simulink library "tqd"  (R2021b)
settings: Solver=VariableStepAuto  StartTime=0.0  StopTime=10.0  RelTol=1e-3
undefined symbols (not defined in the file or in its folder): ATQD_APSDecReq_X_kph, ATQD_APSDecReq_Y_mps2, ATQD_APSDecReqCMD_X_kph, ATQD_APSDecReqTs_X_pct, ATQD_APSDecTimeGain_X_Deg, ATQD_APSDecTimeGain_Y_s, ATQD_APSReqLowSpd_X_Deg, ATQD_AutoHoldReleaseBPS_X_Deg, ATQD_AWDLoadTrqnsGain_X_kg, ATQD_AWDLoadTrqnsGain_Y_pct, ATQD_BOSEnBPSPosn_X_kph, ATQD_BOSMap_X_rpm, ATQD_BOSMap_Y_pct, ATQD_CreepBaseTqD_X_kph, ATQD_CreepBaseTqD_Y_Deg, ATQD_CreepBaseTqR_X_kph, ATQD_CreepBaseTqR_Y_Deg, ATQD_CreepBPSDisPosn_X_Deg, ATQD_CreepBPSDisPosnR_X_Deg, ATQD_CreepBPSEnPosn_X_Deg, ATQD_CreepBPSEnPosnR_X_Deg, ATQD_CreepDeltaTq_X_kph, ATQD_CreepIterm_X_kph, ATQD_CreepIterm_Y_kph, ATQD_CreepItermMaxLimit_X_pct, ATQD_CreepPreloadTime_X_kph, ATQD_CreepPreloadTq_X_kph, ATQD_CreepPreloadTq_Y_s, ATQD_CreepProtTq_X_Deg, ATQD_CreepPterm_X_kph, ATQD_ECOTqMapD_X_rpm, ATQD_ECOTqMapD_Y_pct, ATQD_EOPDTqMapDCon_X_rpm, ATQD_EOPDTqMapDCon_Y_Deg, ATQD_EstInitVehWeight_X_c, ATQD_LHMRollGenMapD_X_rpm, ATQD_LHMRollGenMapD_Y_rpm, ATQD_LHMTqMapD_X_rpm, ATQD_LHMTqMapD_Y_pct, ATQD_NL1TqMapD_X_rpm, ATQD_NL1TqMapD_Y_pct, ATQD_NOPDTqMapDCon_X_rpm, ATQD_NOPDTqMapDCon_Y_Deg, ATQD_NRMRrEDUSpRat_X_rpm, ATQD_NRMRrEDUSpRat_Y_Nm, ATQD_OPDHoldDownRelDelay_X_Deg, ATQD_OPDHoldEnSpd_X_Deg, ATQD_OPDHoldRelDetTime_X_Deg, ATQD_OPDHoldReleaseTq_X_Deg, ATQD_OrigPedTqLowLim_X_Deg, ATQD_OrigPedTqLowLim_Y_pct, ATQD_PedalMapClimbUpLim_X_rpm, ATQD_PedalMapClimbUpLim_Y_Deg, ATQD_PreLoadTq_X_s, ATQD_RollGenMapEL1_X_rpm, ATQD_RollGenMapEL1_Y_rpm, ATQD_SL1TqMapD_X_rpm, ATQD_SL1TqMapD_Y_pct, ATQD_SlideRegenTqGain_X_Gps, ATQD_SlideRegenTqGain_Y_pct ... (+378)
libraries: hcu_lib x59, simulink x49
(part 8 of 12)

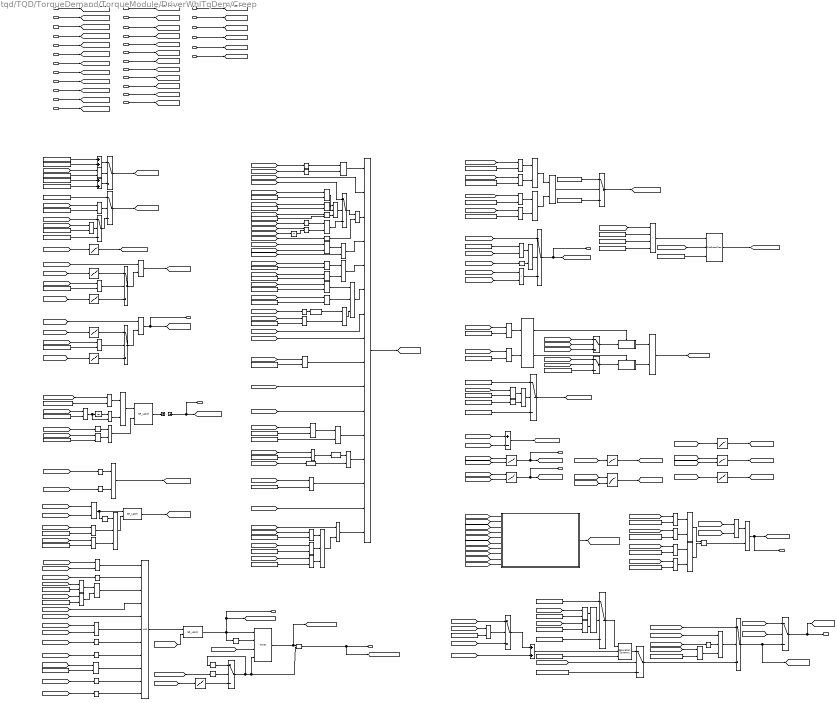
== system tqd/TQD/TorqueDemand/TorqueModule/DriverWhlTqDem/Creep ==
  note: Creep Wheel Torque Demand Calculation
  note: Vehicle Actual Speed Calculation
  note: Creep Enable Judgement
  VTQD_CreepON_flg : Inport
  VTQD_GearActualPosn_enum : Inport  Port=2
  VTQD_LowIdleAccPedal_flg : Inport  Port=3
  VINP_VehSpeed_kph : Inport  Port=4
  VTQD_TMRotateDirction_enum : Inport  Port=5
  VTQD_RegenMode_enum : Inport  Port=6
  VTQD_ActBPSPosn_pct : Inport  Port=7
  VTQD_PedalMapWhlTq_Nm : Inport  Port=8
  VINP_RrRBCActive_flg : Inport  Port=9
  VINP_FrRBCActive_flg : Inport  Port=10
  VVMC_ADASActive_flg : Inport  Port=11
  task_time_s : Inport  Port=12
  VTQD_LoSpdBrkCtrl_flg : Inport  Port=13
  VINP_AVHActive_flg : Inport  Port=14
  VTQD_APSReq_enum : Inport  Port=15
  VVMC_APSSpeedCMD_kph : Inport  Port=16
  VVMC_APSActive_flg : Inport  Port=17
  VTQD_RDCActive_enum : Inport  Port=18
  VVMC_APSReq_enum : Inport  Port=19
  " VINP_FrEDURealTMTq_Nm" : Inport  Port=20
  VINP_RrEDURealTMTq_Nm : Inport  Port=21
  VTQD_PreLoadPreEn_flg : Inport  Port=22
  VVMC_EstSlope_Deg : Inport  Port=23
  VPMM_PwrSta_enum : Inport  Port=24
  VTQD_TqTargetShaftSpd_rpm : Inport  Port=25
  VTQD_APSReqTimer_s : Inport  Port=26
  VINP_EPBSta_enum : Inport  Port=27
  VTQD_OPDHoldEnRel_flg : Inport  Port=28
  VTQD_ActAPSPosn_pct : Inport  Port=29
  VVMC_CAASActive_flg : Inport  Port=30
  AND{,1..2,4..7,9,11..13,15} (12 alike) : Logic  AllPortsSameDT=off  OutDataTypeStr=boolean
  AND10 : Logic  Operator=OR  AllPortsSameDT=off  OutDataTypeStr=boolean
  AND14 : Logic  Inputs=3  AllPortsSameDT=off  OutDataTypeStr=boolean
  AND3 : Logic  Inputs=3  AllPortsSameDT=off  OutDataTypeStr=boolean
  AND8 : Logic  Inputs=3  AllPortsSameDT=off  OutDataTypeStr=boolean
  Add : Sum  Inputs=+-
  Add1 : Sum
  Add2 : Sum
  Add4 : Sum
  Constant1 : Constant  Value=KTQD_APSCMDEnCreepSpd_kph
  Constant10 : Constant  Value=KTQD_CreepTargetSpdR_kph
  Constant{3,11..12,21,25,58,62} (7 alike) : Constant  Value=ENUM_GEARACTUALPOSN_D
  Constant13 : Constant  Value=KTQD_CreepEnableSpd_kph
  Constant14 : Constant  Value=RPM2RADPS
  Constant15 : Constant  Value=ZERO_FLOAT
  Constant16 : Constant  Value=KTQD_TireRadius_m
  Constant17 : Constant  Value=ENUM_RDCACTSTA_NOREQUEST
  Constant18 : Constant  Value=ENUM_APSREQ_DECELCTRL  OutDataTypeStr=uint8
  Constant19 : Constant  Value=MPS2KPH
  Constant{2,9,20,31,35..36,38,42..44} (10 alike) : Constant  Value=ENUM_GEARACTUALPOSN_R
  Constant22 : Constant  Value=KTQD_CreepLowLimitTq_Nm
  Constant23 : Constant  Value=KTQD_CreepPrLoadEnSpd_kph
  Constant24 : Constant  Value=ENUM_RDCACTSTA_NOREQUEST
  Constant26 : Constant  Value=KTQD_CreepDisableSpdofst_kph
  Constant27 : Constant  Value=KTQD_CreepEnableSpdR_kph
  Constant28 : Constant  Value=KTQD_CreepDisableSpdofstR_kph
  Constant29 : Constant  Value=KTQD_CreepEnableSpdR_kph
  Constant30 : Constant  Value=ENUM_TMROTATEDIRECTACT_REVERSE  OutDataTypeStr=Inherit: Inherit via back propagation
  Constant32 : Constant  Value=ENUM_TMROTATEDIRECTACT_FORWARD  OutDataTypeStr=Inherit: Inherit via back propagation
  Constant33 : Constant  Value=KTQD_VehActSpdNegGain_gain
  Constant34 : Constant  Value=KTQD_VehActSpdPosGain_gain
  Constant37 : Constant  Value=ENUM_TMROTATEDIRECTACT_REVERSE  OutDataTypeStr=Inherit: Inherit via back propagation
  Constant39 : Constant  Value=ENUM_TMROTATEDIRECTACT_FORWARD  OutDataTypeStr=Inherit: Inherit via back propagation
  Constant{4,8,52,54,59,64} (6 alike) : Constant  Value=ENUM_REGENLEVEL_OPD
  Constant40 : Constant  Value=KTQD_RBCCreepRecTq_Nm
  Constant41 : Constant  Value=KTQD_RBCCreepRecTq_Nm
  Constant45 : Constant  Value=ENUM_POWERSTA_READY
  Constant46 : Constant  Value=KTQD_CreepEnableSpd_kph
  Constant47 : Constant  Value=KTQD_RPM2VehSpdTs_c
  Constant48 : Constant  Value=KTQD_CreepVehSpdSW_flg
  Constant49 : Constant  Value=KTQD_CreepTargetSpdD_kph
  Constant5 : Constant  Value=ENUM_APSREQ_BRKHOLD  OutDataTypeStr=uint8
  Constant50 : Constant  Value=KTQD_OPDCreepTargetSpdD_kph
  Constant51 : Constant  Value=KTQD_APSReqDisCreep_flg  OutDataTypeStr=uint8
  Constant53 : Constant  Value=KTQD_APSReqDelayTime_s
  Constant55 : Constant  Value=ENUM_EPBSTA_APPLIED  OutDataTypeStr=uint8
  Constant56 : Constant  Value=KTQD_APSReqDisCreep_flg
  Constant57 : Constant  Value=KTQD_CreepUpLimitTq_Nm
  Constant6 : Constant  Value=ENUM_GEARACTUALPOSN_P
  Constant60 : Constant  Value=KTQD_OPDCreepDUpLimitTq_Nm
  Constant61 : Constant  Value=KTQD_CreepDisPedTqSpd_kph
  Constant63 : Constant  Value=KTQD_CreepAPSPosn2Launch_pct
  Constant65 : Constant  Value=ENUM_APSREQ_DECELCTRL  OutDataTypeStr=uint8
  Constant7 : Constant  Value=ENUM_GEARACTUALPOSN_N
  Data Type Conversion : DataTypeConversion
  Delay : Delay  DelayLength=1
  Delay1 : Delay  DelayLength=1
  Detect Change : simulink/Logic and Bit Operations/Detect Change  vinit=0  OutDataTypeStr=boolean
  Detect Increase : simulink/Logic and Bit Operations/Detect Increase  vinit=0.0  OutDataTypeStr=boolean
  Equal{,1..4,6..8,10..16,19..31,33..39} (35 alike) : RelationalOperator  Operator===  OutDataTypeStr=boolean  RndMeth=Simplest
  Equal17 : RelationalOperator  Operator=<=  OutDataTypeStr=boolean  RndMeth=Simplest
  Equal18 : RelationalOperator  Operator=~=  OutDataTypeStr=boolean  RndMeth=Simplest
  Equal32 : RelationalOperator  OutDataTypeStr=boolean  RndMeth=Simplest
  Equal5 : RelationalOperator  Operator=<=  OutDataTypeStr=boolean  RndMeth=Simplest
  Equal9 : RelationalOperator  Operator=<=  OutDataTypeStr=boolean  RndMeth=Simplest
  FirstOrderFilter : hcu_lib/Basic_Blocks/FirstOrderFilter
  GreaterThan : RelationalOperator  Operator=>  OutDataTypeStr=boolean  RndMeth=Simplest
  GreaterThan1 : RelationalOperator  Operator=>  OutDataTypeStr=boolean  RndMeth=Simplest
  GreaterThan2 : RelationalOperator  OutDataTypeStr=boolean  RndMeth=Simplest
  GreaterThan3 : RelationalOperator  Operator=>  OutDataTypeStr=boolean  RndMeth=Simplest
  GreaterThan4 : RelationalOperator  Operator=<=  OutDataTypeStr=boolean  RndMeth=Simplest
  Ground2 : Ground
  If : If  NumInputs=2  IfExpression=u1 ~= 0  ElseIfExpressions=u2 ~= 0  ShowElse=off
  If Action Subsystem : Subsystem  TreatAsAtomicUnit=on
  If Action Subsystem1 : Subsystem  TreatAsAtomicUnit=on
  LiuzgSwitch1 : Switch  Criteria=u2 ~= 0
      settings: AttributesFormatString=<%<Criteria>>
  Logical Operator{,2,4,6} (4 alike) : Logic  AllPortsSameDT=off  OutDataTypeStr=boolean
  Logical Operator1 : Logic  Operator=OR  AllPortsSameDT=off  OutDataTypeStr=boolean
  Logical Operator3 : Logic  Inputs=11  AllPortsSameDT=off  OutDataTypeStr=boolean
  Logical Operator5 : Logic  Operator=OR  AllPortsSameDT=off  OutDataTypeStr=boolean
  MTQD_CreepBPSDisPosnR_Y_pct : Lookup_n-D  NumberOfTableDimensions=1  BreakpointsForDimension1=ATQD_CreepBPSDisPosnR_X_Deg  Table=MTQD_CreepBPSDisPosnR_Y_pct  ExtrapMethod=Clip  InternalRulePriority=Speed  RndMeth=Simplest  InputSameDT=on
  MTQD_CreepBPSDisPosn_Y_pct : Lookup_n-D  NumberOfTableDimensions=1  BreakpointsForDimension1=ATQD_CreepBPSDisPosn_X_Deg  Table=MTQD_CreepBPSDisPosn_Y_pct  ExtrapMethod=Clip  InternalRulePriority=Speed  RndMeth=Simplest  InputSameDT=on
  MTQD_CreepBPSEnPosnR_Y_pct : Lookup_n-D  NumberOfTableDimensions=1  BreakpointsForDimension1=ATQD_CreepBPSEnPosnR_X_Deg  Table=MTQD_CreepBPSEnPosnR_Y_pct  ExtrapMethod=Clip  InternalRulePriority=Speed  RndMeth=Simplest  InputSameDT=on
  MTQD_CreepBPSEnPosn_Y_pct : Lookup_n-D  NumberOfTableDimensions=1  BreakpointsForDimension1=ATQD_CreepBPSEnPosn_X_Deg  Table=MTQD_CreepBPSEnPosn_Y_pct  ExtrapMethod=Clip  InternalRulePriority=Speed  RndMeth=Simplest  InputSameDT=on
  MTQD_CreepBaseTqD_Z_Nm : Lookup_n-D  BreakpointsForDimension1=ATQD_CreepBaseTqD_Y_Deg  BreakpointsForDimension2=ATQD_CreepBaseTqD_X_kph  Table=MTQD_CreepBaseTqD_Z_Nm  ExtrapMethod=Clip  InternalRulePriority=Speed  RndMeth=Simplest  InputSameDT=on
      settings: InputPortMap=u0,u1
  MTQD_CreepBaseTqR_Z_Nm : Lookup_n-D  BreakpointsForDimension1=ATQD_CreepBaseTqR_Y_Deg  BreakpointsForDimension2=ATQD_CreepBaseTqR_X_kph  Table=MTQD_CreepBaseTqR_Z_Nm  ExtrapMethod=Clip  InternalRulePriority=Speed  RndMeth=Simplest  InputSameDT=on
      settings: InputPortMap=u0,u1
  MTQD_CreepDeltaTq_Y_Nm : Lookup_n-D  NumberOfTableDimensions=1  BreakpointsForDimension1=ATQD_CreepDeltaTq_X_kph  Table=MTQD_CreepDeltaTq_Y_Nm  ExtrapMethod=Clip  InternalRulePriority=Speed  RndMeth=Simplest  InputSameDT=on
  MTQD_CreepIterm_Z_Nm : Lookup_n-D  BreakpointsForDimension1=ATQD_CreepIterm_Y_kph  BreakpointsForDimension2=ATQD_CreepIterm_X_kph  Table=MTQD_CreepIterm_Z_Nm  ExtrapMethod=Clip  InternalRulePriority=Speed  RndMeth=Simplest  InputSameDT=on
      settings: InputPortMap=u0,u1
  MTQD_CreepPrelaodTq_Z_Nm : Lookup_n-D  BreakpointsForDimension1=ATQD_CreepPreloadTq_Y_s  BreakpointsForDimension2=ATQD_CreepPreloadTq_X_kph  Table=MTQD_CreepPreloadTq_Z_Nm  ExtrapMethod=Clip  InternalRulePriority=Speed  RndMeth=Simplest  InputSameDT=on
      settings: InputPortMap=u0,u1
  MTQD_CreepPreloadTime_Y_s : Lookup_n-D  NumberOfTableDimensions=1  BreakpointsForDimension1=ATQD_CreepPreloadTime_X_kph  Table=MTQD_CreepPreloadTime_Y_s  ExtrapMethod=Clip  InternalRulePriority=Speed  RndMeth=Simplest  InputSameDT=on
  MTQD_CreepProtTq_Y_Nm : Lookup_n-D  NumberOfTableDimensions=1  BreakpointsForDimension1=ATQD_CreepProtTq_X_Deg  Table=MTQD_CreepProtTq_Y_Nm  ExtrapMethod=Clip  InternalRulePriority=Speed  RndMeth=Simplest  InputSameDT=on
  MTQD_CreepPterm_Y_c : Lookup_n-D  NumberOfTableDimensions=1  BreakpointsForDimension1=ATQD_CreepPterm_X_kph  Table=MTQD_CreepPterm_Y_Nm  ExtrapMethod=Clip  InternalRulePriority=Speed  RndMeth=Simplest  InputSameDT=on
  MTQD_OPDHoldEnSpd_Y_kph : Lookup_n-D  NumberOfTableDimensions=1  BreakpointsForDimension1=ATQD_OPDHoldEnSpd_X_Deg  Table=MTQD_OPDHoldEnSpd_Y_kph  ExtrapMethod=Clip  InternalRulePriority=Speed  RndMeth=Simplest  InputSameDT=on
  Merge : Merge
  NOT{,1..15} (16 alike) : Logic  Operator=NOT  AllPortsSameDT=off  OutDataTypeStr=boolean
  OR{,2..3,6..9} (7 alike) : Logic  Operator=OR  AllPortsSameDT=off  OutDataTypeStr=boolean
  OR1 : Logic  Operator=OR  Inputs=16  AllPortsSameDT=off  OutDataTypeStr=boolean
  OR4 : Logic  Inputs=3  AllPortsSameDT=off  OutDataTypeStr=boolean
  OR5 : Logic  Operator=OR  Inputs=3  AllPortsSameDT=off  OutDataTypeStr=boolean
  Product : Product
  Product1 : Product  Inputs=4
  Relational Operator : RelationalOperator  OutDataTypeStr=boolean  RndMeth=Simplest
  Relational Operator1 : RelationalOperator  Operator=<  OutDataTypeStr=boolean  RndMeth=Simplest
  Relational Operator2 : RelationalOperator  Operator=>  OutDataTypeStr=boolean  RndMeth=Simplest
  Relational Operator3 : RelationalOperator  Operator=>  OutDataTypeStr=boolean  RndMeth=Simplest
  Relational Operator4 : RelationalOperator  Operator=>  OutDataTypeStr=boolean  RndMeth=Simplest
  Relational Operator5 : RelationalOperator  Operator=<=  OutDataTypeStr=boolean  RndMeth=Simplest
  Relay : Relay  OnSwitchValue=KTQD_OPDCreepEnGrade_Deg  OffSwitchValue=KTQD_OPDCreepDisGrade_Deg  OnOutputValue=0  OffOutputValue=1
  Relay1 : Relay  OnSwitchValue=KTQD_CreepDisVehSpd_kph  OffSwitchValue=KTQD_CreepEnVehSpd_kph  OnOutputValue=0  OffOutputValue=1  OutDataTypeStr=boolean
  SR_Latch : hcu_lib/Basic_Blocks/SR_Latch
  SR_Latch1 : hcu_lib/Basic_Blocks/SR_Latch
  SR_Latch3 : hcu_lib/Basic_Blocks/SR_Latch
  Saturation Dynamic : simulink/Discontinuities/Saturation Dynamic  OutMin=[]  OutMax=[]  OutDataTypeStr=Inherit: Same as second input  OutDataType=fixdt(1, 16)  OutScaling=2^-10  DoSatur=off
  Switch{,1..4,7} (6 alike) : Switch  Criteria=u2 ~= 0
  Switch Case Action Subsystem : Subsystem  TreatAsAtomicUnit=on
  Switch{5..6,8..15} (10 alike) : Switch  Criteria=u2 > Threshold
  Terminator3 : Terminator
  Timer : hcu_lib/Basic_Blocks/Timer
  Unit Delay : UnitDelay  SampleTime=-1  HasFrameUpgradeWarning=on
  Unit Delay1 : UnitDelay  SampleTime=-1  HasFrameUpgradeWarning=on
  VTQD_CreepEnable_flg : Outport
  VTQD_CreepWhlTqDem_Nm : Outport  Port=2
  VTQD_CreepPrLoadEnable_flg : Outport  Port=3
  VTQD_OPDOn2Off_flg : Outport  Port=4
  VTQD_CreepProtTqEn_flg : Outport  Port=5
  VTQD_VehActSpd_kph : Outport  Port=6
  VTQD_CreepBaseTqD_Nm : Outport  Port=7
  VTQD_CreepBaseTqR_Nm : Outport  Port=8
  VTQD_HighBPSPosn_flg : Outport  Port=9
  wires:
  Equal37/1 -> AND14/1
  GreaterThan4/1 -> AND14/2
  AND14/1 -> Switch15/2
  Constant62/1 -> Equal37/2
  [VTQD_GearActualPosn_enum] -> Equal37/1
  [VTQD_OPDHoldEnRel_flg] -> Switch15/1
  VTQD_OPDHoldEnRel_flg/1 -> [VTQD_OPDHoldEnRel_flg]
  Switch15/1 -> AND1/1
  NOT1/1 -> AND1/2
  Constant61/1 -> GreaterThan4/2
  [VTQD_VehActSpd_kph] -> GreaterThan4/1
  VTQD_APSReqTimer_s/1 -> [VTQD_APSReqTimer_s]
  VTQD_TqTargetShaftSpd_rpm/1 -> [VTQD_TqTargetShaftSpd_rpm]
  VINP_EPBSta_enum/1 -> [VINP_EPBSta_enum]
  Saturation Dynamic/1 -> Switch/1
  Constant57/1 -> Switch14/3
  Equal36/1 -> AND13/2
  [VTQD_RegenMode_enum] -> Equal36/1
  Equal35/1 -> AND13/1
  AND13/1 -> Switch14/2
  Constant58/1 -> Equal35/2
  [VTQD_GearActualPosn_enum] -> Equal35/1
  Switch14/1 -> Saturation Dynamic/1  "VTQD_CreepUpLimitTq_Nm"
  Constant59/1 -> Equal36/2
  Constant60/1 -> Switch14/1
  Constant22/1 -> Saturation Dynamic/3
  Add2/1 -> Saturation Dynamic/2
  Constant50/1 -> Switch12/1
  Constant52/1 -> Equal31/2
  [VTQD_RegenMode_enum] -> Equal31/1
  NOT14/1 -> AND12/2
  Constant56/1 -> NOT14/1
  Switch12/1 -> [VTQD_CreepTargetSpdD_kph]  "VTQD_CreepTargetSpdD_kph"
  AND12/1 -> Switch12/2
  Equal31/1 -> AND12/1
  Constant49/1 -> Switch12/3
  [VTQD_TqTargetShaftSpd_rpm] -> Product1/1
  [VINP_VehSpeed_kph] -> Relay1/1
  AND10/1 -> AND9/1
  [task_time_s] -> FirstOrderFilter/2
  Relay1/1 -> AND9/2
  [VVMC_APSActive_flg] -> AND10/2
  Constant14/1 -> Product1/2
  [VINP_VehSpeed_kph] -> Product/2
  Product/1 -> Switch11/3
  [VTQD_RPM2VehSpd_kph] -> Switch11/1
  AND9/1 -> Switch11/2
  Product1/1 -> FirstOrderFilter/1
  FirstOrderFilter/1 -> [VTQD_RPM2VehSpd_kph]  "VTQD_RPM2VehSpd_kph"
  Switch11/1 -> [VTQD_VehActSpd_kph], VTQD_VehActSpd_kph/1  "VTQD_VehActSpd_kph"
  Constant47/1 -> FirstOrderFilter/3
  Constant48/1 -> AND10/1
  [VTQD_VehActSpdGain_gain] -> Product/1
  Constant19/1 -> Product1/4
  Constant16/1 -> Product1/3
  [VINP_EPBSta_enum] -> Equal34/1
  Constant55/1 -> Equal34/2
  Equal34/1 -> OR1/14
  AND11/1 -> OR1/12
  Constant51/1 -> AND11/2
  Equal15/1 -> AND11/1
  Constant18/1 -> Equal15/2
  [VTQD_APSReq_enum] -> Equal15/1
  OR8/1 -> OR4/3
  Data Type Conversion/1 -> OR8/1  "VTQD_OPDCreepGrade_flg"
  Equal32/1 -> OR8/2
  [VTQD_APSReqTimer_s] -> Equal32/1
  Constant53/1 -> Equal32/2
  [VTQD_RBCActive_flg] -> OR1/7
  OR4/1 -> OR1/6
  NOT13/1 -> AND6/2
  NOT12/1 -> AND6/1
  [VTQD_HighBPSPosn_flg] -> NOT13/1
  [VTQD_LowBPSPosn_flg] -> NOT12/1
  MTQD_OPDHoldEnSpd_Y_kph/1 -> [VTQD_OPDHoldEnSpd_kph]  "VTQD_OPDHoldEnSpd_kph"
  [VVMC_EstSlope_Deg] -> MTQD_OPDHoldEnSpd_Y_kph/1
  Switch13/1 -> Switch6/3
  Equal33/1 -> Switch13/2
  Constant54/1 -> Equal33/2
  [VTQD_RegenMode_enum] -> Equal33/1
  [VTQD_OPDHoldEnSpd_kph] -> Switch13/1
  Constant46/1 -> Switch13/3
  [VTQD_GearActualPosn_enum] -> Detect Change/1
  [VVMC_EstSlope_Deg] -> MTQD_CreepProtTq_Y_Nm/1
  [VTQD_CreepErrSpd_kph] -> MTQD_CreepDeltaTq_Y_Nm/1
  MTQD_CreepProtTq_Y_Nm/1 -> [VTQD_CreepProtTq_Nm]  "VTQD_CreepProtTq_Nm"
  MTQD_CreepPrelaodTq_Z_Nm/1 -> [VTQD_CreepPreloadTq_Nm]  "VTQD_CreepPreloadTq_Nm"
  [VVMC_EstSlope_Deg] -> MTQD_CreepBaseTqD_Z_Nm/1
  [VTQD_CreepFinalSpd_kph] -> Add/1
  MTQD_CreepBaseTqR_Z_Nm/1 -> [VTQD_CreepBaseTqR_Nm], VTQD_CreepBaseTqR_Nm/1  "VTQD_CreepBaseTqR_Nm"
  [VTQD_CreepPreloadTime_s] -> MTQD_CreepPrelaodTq_Z_Nm/1
  [VTQD_VehActSpd_kph] -> MTQD_CreepBaseTqR_Z_Nm/2
  [VTQD_VehActSpd_kph] -> Add/2
  [VTQD_CreepErrSpd_kph] -> MTQD_CreepPterm_Y_c/1
  MTQD_CreepDeltaTq_Y_Nm/1 -> [VTQD_CreepDeltaTq_Nm]  "VTQD_CreepDeltaTq_Nm"
  [VTQD_VehActSpd_kph] -> MTQD_CreepBaseTqD_Z_Nm/2
  MTQD_CreepBaseTqD_Z_Nm/1 -> [VTQD_CreepBaseTqD_Nm], VTQD_CreepBaseTqD_Nm/1  "VTQD_CreepBaseTqD_Nm"
  [VVMC_EstSlope_Deg] -> MTQD_CreepBaseTqR_Z_Nm/1
  [VINP_VehSpeed_kph] -> MTQD_CreepPrelaodTq_Z_Nm/2
  Add/1 -> [VTQD_CreepErrSpd_kph]  "VTQD_CreepErrSpd_kph"
  MTQD_CreepPterm_Y_c/1 -> [VTQD_CreepPterm_c]  "VTQD_CreepPterm_c"
  Switch10/1 -> Timer/4, Relational Operator/2, Delay/1
  MTQD_CreepPreloadTime_Y_s/1 -> Switch10/3  "VTQD_CreepPreloadSetTime_s"
  Delay1/1 -> Switch10/2
  [VTQD_CreepEnable_flg] -> Delay1/1
  Delay/1 -> Switch10/1
  [VTQD_PreLoadPreEn_flg] -> NOT11/1
  NOT11/1 -> Logical Operator3/11
  [VVMC_EstSlope_Deg] -> MTQD_CreepBPSEnPosn_Y_pct/1
  [VTQD_ActBPSPosn_pct] -> Equal5/1
  MTQD_CreepBPSEnPosnR_Y_pct/1 -> Switch8/1  "VTQD_CreepBPSEnPosnR_pct"
  [VTQD_GearActualPosn_enum] -> Equal27/1
  MTQD_CreepBPSDisPosnR_Y_pct/1 -> Switch9/1  "VTQD_CreepBPSDisPosnR_pct"
  MTQD_CreepBPSEnPosn_Y_pct/1 -> Switch8/3  "VTQD_CreepBPSEnPosn_pct"
  [VVMC_EstSlope_Deg] -> MTQD_CreepBPSEnPosnR_Y_pct/1
  Switch8/1 -> Equal5/2
  Constant42/1 -> Equal27/2
  [VTQD_GearActualPosn_enum] -> Equal28/1
  [VVMC_EstSlope_Deg] -> MTQD_CreepBPSDisPosn_Y_pct/1
  Equal28/1 -> Switch9/2
  Equal5/1 -> [VTQD_LowBPSPosn_flg]  "VTQD_LowBPSPosn_flg"
  Switch9/1 -> GreaterThan2/2
  GreaterThan2/1 -> VTQD_HighBPSPosn_flg/1, [VTQD_HighBPSPosn_flg]  "VTQD_HighBPSPosn_flg"
  [VTQD_ActBPSPosn_pct] -> GreaterThan2/1
  MTQD_CreepBPSDisPosn_Y_pct/1 -> Switch9/3  "VTQD_CreepBPSDisPosn_pct"
  Equal27/1 -> Switch8/2
  [VVMC_EstSlope_Deg] -> MTQD_CreepBPSDisPosnR_Y_pct/1
  Constant43/1 -> Equal28/2
  AND4/1 -> SR_Latch3/1
  Unit Delay1/1 -> GreaterThan3/1
  OR2/1 -> SR_Latch3/2
  [VTQD_RegenMode_enum] -> Equal4/1
  NOT6/1 -> OR2/1
  Constant44/1 -> Equal29/2
  Constant45/1 -> Equal30/2
  Equal30/1 -> AND4/1
  GreaterThan3/1 -> AND4/2
  [VTQD_LowIdleAccPedal_flg] -> NOT6/1
  Constant4/1 -> Equal4/2
  Equal4/1 -> Unit Delay1/1, GreaterThan3/2
  [VTQD_GearActualPosn_enum] -> Equal29/1
  Equal29/1 -> OR2/2
  [VPMM_PwrSta_enum] -> Equal30/1
  VPMM_PwrSta_enum/1 -> [VPMM_PwrSta_enum]
  VVMC_EstSlope_Deg/1 -> [VVMC_EstSlope_Deg]
  VTQD_PreLoadPreEn_flg/1 -> [VTQD_PreLoadPreEn_flg]
  Ground2/1 -> VTQD_OPDOn2Off_flg/1, [VTQD_OPDOn2Off_flg]  "VTQD_OPDOn2Off_flg"
  Relay/1 -> Data Type Conversion/1
  [VVMC_EstSlope_Deg] -> Relay/1
  " VINP_FrEDURealTMTq_Nm"/1 -> [VINP_FrEDURealTMTq_Nm]
  VINP_RrEDURealTMTq_Nm/1 -> [VINP_RrEDURealTMTq_Nm]
  [VINP_FrRBCActive_flg] -> OR7/2
  [VINP_RrRBCActive_flg] -> OR7/1
  Relational Operator3/1 -> AND8/3
  [VINP_RrEDURealTMTq_Nm] -> Relational Operator3/1
  Constant40/1 -> Relational Operator3/2
  [VINP_FrEDURealTMTq_Nm] -> Relational Operator4/1
  OR7/1 -> SR_Latch1/1, NOT7/1
  Constant41/1 -> Relational Operator4/2
  AND8/1 -> SR_Latch1/2  "VTQD_RBCActiveRec_flg"
  SR_Latch1/1 -> [VTQD_RBCActive_flg]  "VTQD_RBCActive_flg"
  NOT7/1 -> AND8/1
  Relational Operator4/1 -> AND8/2
  [VTQD_CreepProtTq_Nm] -> Switch7/1
  Switch7/1 -> [VTQD_CreepWhlTqDem_Nm], VTQD_CreepWhlTqDem_Nm/1  "VTQD_CreepWhlTqDem_Nm"
  [VTQD_CreepProtTqEn_flg] -> Switch7/2
  Switch4/1 -> Switch7/3, [VTQD_CreepActWhlTqDem_Nm]  "VTQD_CreepActWhlTqDem_Nm"
  Logical Operator6/1 -> OR6/2
  Equal26/1 -> Logical Operator6/2
  OR6/1 -> AND7/2
  Constant37/1 -> Equal24/2
  Equal24/1 -> Logical Operator4/2
  Equal23/1 -> Logical Operator4/1
  Constant11/1 -> Equal23/2
  [VTQD_TMRotateDirction_enum] -> Equal24/1
  [VTQD_GearActualPosn_enum] -> Equal23/1
  Logical Operator4/1 -> OR6/1
  Constant39/1 -> Equal26/2
  [VTQD_TMRotateDirction_enum] -> Equal26/1
  [VTQD_CreepActWhlTqDem_Nm] -> Relational Operator2/2
  Relational Operator2/1 -> AND7/1
  Constant38/1 -> Equal25/2
  [VTQD_CreepProtTq_Nm] -> Relational Operator2/1
  [VTQD_GearActualPosn_enum] -> Equal25/1
  Equal25/1 -> Logical Operator6/1
  AND7/1 -> [VTQD_CreepProtTqEn_flg], VTQD_CreepProtTqEn_flg/1  "VTQD_CreepProtTqEn_flg"
  Constant28/1 -> Add1/2
  Constant26/1 -> Add4/2
  Constant13/1 -> Add4/1
  Add4/1 -> Switch5/3
  Constant27/1 -> Add1/1
  Equal21/1 -> Switch5/2
  [VTQD_GearActualPosn_enum] -> Equal21/1
  Add1/1 -> Switch5/1
  [VTQD_GearActualPosn_enum] -> Equal22/1
  Constant35/1 -> Equal21/2
  Switch5/1 -> [VTQD_CreepDisSpd_kph]  "VTQD_CreepDisSpd_kph"
  Constant36/1 -> Equal22/2
  Switch6/1 -> [VTQD_CreepEnSpd_kph]  "VTQD_CreepEnSpd_kph"
  Constant29/1 -> Switch6/1
  Equal22/1 -> Switch6/2
  VVMC_APSReq_enum/1 -> [VVMC_APSReq_enum]
  Equal19/1 -> OR4/2
  Constant25/1 -> Equal19/2
  [VTQD_GearActualPosn_enum] -> Equal19/1
  Equal11/1 -> OR4/1
  [VINP_AVHActive_flg] -> OR1/11
  Equal18/1 -> OR1/9
  [VTQD_RDCActive_enum] -> Equal18/1
  Constant24/1 -> Equal18/2
  Constant17/1 -> Equal14/2
  [VTQD_RDCActive_enum] -> Equal14/1
  VTQD_RDCActive_enum/1 -> [VTQD_RDCActive_enum]
  [VTQD_LoSpdBrkCtrl_flg] -> OR1/10
  [VVMC_ADASActive_flg] -> OR1/8
  OR/1 -> OR1/5
  AND2/1 -> OR1/4
  AND1/1 -> OR1/3
  Equal17/1 -> AND3/3
  Constant23/1 -> Equal17/2
  [VINP_VehSpeed_kph] -> Equal17/1
  [VTQD_OPDOn2Off_flg] -> If Action Subsystem1/10(VTQD_OPDOn2Off)
  AND3/1 -> Switch4/2
  [VTQD_CreepPrLoadEnable_flg] -> AND3/1
  [VTQD_CreepPreloadTq_Nm] -> Switch4/1
  NOT10/1 -> AND3/2
  [VTQD_CreepEnable_flg] -> NOT10/1
  NOT8/1 -> Timer/2
  SR_Latch/1 -> Timer/1, NOT8/1, [VTQD_CreepPrLoadEnable_flg], VTQD_CreepPrLoadEnable_flg/1  "VTQD_CreepPrLoadEnable_flg"
  Relational Operator/1 -> VTQD_CreepEnable_flg/1, [VTQD_CreepEnable_flg]  "VTQD_CreepEnable_flg"
  [task_time_s] -> Timer/3
  Timer/1 -> Relational Operator/1, [VTQD_CreepPreloadTime_s]  "VTQD_CreepPreloadTime_s"
  Equal16/1 -> Switch3/2
  [VTQD_GearActualPosn_enum] -> Equal16/1
  Constant9/1 -> Equal16/2
  Switch3/1 -> Add2/1  "VTQD_ActCreepBaseTq_Nm"
  [VTQD_CreepBaseTqR_Nm] -> Switch3/1
  [VTQD_CreepBaseTqD_Nm] -> Switch3/3
  NOT5/1 -> AND/1
  [VVMC_APSActive_flg] -> NOT5/1
  AND/1 -> OR1/1
  NOT2/1 -> AND/2
  OR3/1 -> Logical Operator3/1
  [VTQD_CreepON_flg] -> OR3/2
  [VVMC_APSActive_flg] -> OR3/1
  Constant10/1 -> Switch2/3
  Switch2/1 -> Switch Case Action Subsystem/1(In1)
  [VVMC_APSActive_flg] -> Switch2/2
  [VVMC_APSActive_flg] -> Switch1/2
  [VTQD_CreepTargetSpdD_kph] -> Switch1/3
  Switch1/1 -> If Action Subsystem/1(In1)
  VVMC_APSActive_flg/1 -> [VVMC_APSActive_flg]
  VVMC_APSSpeedCMD_kph/1 -> [VVMC_APSSpeedCMD_kph]
  VTQD_APSReq_enum/1 -> [VTQD_APSReq_enum]
  VINP_AVHActive_flg/1 -> [VINP_AVHActive_flg]
  [VTQD_CreepDisable_flg] -> If Action Subsystem1/8(VTQD_CreepDisable_flg)
  VTQD_LoSpdBrkCtrl_flg/1 -> [VTQD_LoSpdBrkCtrl_flg]
  NOT9/1 -> Logical Operator3/10
  [VTQD_LoSpdBrkCtrl_flg] -> NOT9/1
  Constant15/1 -> Switch/3
  [VTQD_CreepEnable_flg] -> Switch/2
  Switch/1 -> Switch4/3
  Equal14/1 -> Logical Operator3/9
  SR_Latch3/1 -> Terminator3/1
  VINP_VehSpeed_kph/1 -> [VINP_VehSpeed_kph]
  VTQD_GearActualPosn_enum/1 -> [VTQD_GearActualPosn_enum]
  Logical Operator3/1 -> SR_Latch/1
  VTQD_CreepON_flg/1 -> [VTQD_CreepON_flg]
  VTQD_LowIdleAccPedal_flg/1 -> [VTQD_LowIdleAccPedal_flg]
  Constant32/1 -> Equal3/2
  [VTQD_TMRotateDirction_enum] -> Equal3/1
  [VTQD_GearActualPosn_enum] -> Equal2/1
  Logical Operator/1 -> Logical Operator1/1
  Logical Operator1/1 -> LiuzgSwitch1/2
  Logical Operator2/1 -> Logical Operator1/2
  Equal2/1 -> Logical Operator2/1
  Constant31/1 -> Equal2/2
  Equal1/1 -> Logical Operator/2
  Constant30/1 -> Equal1/2
  Equal3/1 -> Logical Operator2/2
  LiuzgSwitch1/1 -> [VTQD_VehActSpdGain_gain]  "VTQD_VehActSpdGain_gain"
  [VTQD_GearActualPosn_enum] -> Equal/1
  Equal/1 -> Logical Operator/1
  Constant3/1 -> Equal/2
  [VTQD_TMRotateDirction_enum] -> Equal1/1
  VTQD_TMRotateDirction_enum/1 -> [VTQD_TMRotateDirction_enum]
  Constant33/1 -> LiuzgSwitch1/1
  Constant34/1 -> LiuzgSwitch1/3
  VTQD_RegenMode_enum/1 -> [VTQD_RegenMode_enum]
  Equal9/1 -> Logical Operator3/6
  Logical Operator5/1 -> Logical Operator3/3
  [VTQD_VehActSpd_kph] -> Equal9/1
  [VTQD_LowIdleAccPedal_flg] -> Logical Operator3/5
  [VTQD_GearActualPosn_enum] -> Equal7/1
  Constant21/1 -> Equal8/2
  Constant20/1 -> Equal7/2
  Equal8/1 -> Logical Operator5/2
  [VTQD_GearActualPosn_enum] -> Equal8/1
  Equal7/1 -> Logical Operator5/1
  VTQD_ActBPSPosn_pct/1 -> [VTQD_ActBPSPosn_pct]
  [VTQD_LowBPSPosn_flg] -> Logical Operator3/4
  VTQD_PedalMapWhlTq_Nm/1 -> [VTQD_PedalMapWhlTq_Nm]
  [VTQD_VehActSpd_kph] -> GreaterThan1/1
  [VTQD_CreepDisSpd_kph] -> GreaterThan1/2
  GreaterThan1/1 -> AND2/1
  [VTQD_LowIdleAccPedal_flg] -> AND2/2
  [VTQD_LowIdleAccPedal_flg] -> NOT1/1
  [VTQD_GearActualPosn_enum] -> Equal6/1
  Constant6/1 -> Equal6/2
  [VTQD_GearActualPosn_enum] -> Equal10/1
  Constant7/1 -> Equal10/2
  Equal6/1 -> OR/1
  Equal10/1 -> OR/2
  [VTQD_CreepON_flg] -> NOT2/1
  Constant8/1 -> Equal11/2
  [VTQD_RegenMode_enum] -> Equal11/1
  [VTQD_CreepDisable_flg] -> SR_Latch/2
  OR1/1 -> [VTQD_CreepDisable_flg]  "VTQD_CreepDisable_flg"
  VINP_RrRBCActive_flg/1 -> [VINP_RrRBCActive_flg]
  VINP_FrRBCActive_flg/1 -> [VINP_FrRBCActive_flg]
  VVMC_ADASActive_flg/1 -> [VVMC_ADASActive_flg]
  [VTQD_CreepEnSpd_kph] -> Equal9/2
  [VTQD_RBCActive_flg] -> NOT/1
  [VVMC_ADASActive_flg] -> NOT3/1
  [VTQD_HighBPSPosn_flg] -> OR1/2
  [VTQD_GearActualPosn_enum] -> Equal13/1
  Constant12/1 -> Equal13/2
  Equal13/1 -> If/1
  [VTQD_GearActualPosn_enum] -> Equal12/1
  Constant2/1 -> Equal12/2
  Equal12/1 -> If/2
  If/1 -> If Action Subsystem/Action
  If/2 -> Switch Case Action Subsystem/Action
  If Action Subsystem/1(Out1) -> Merge/1
  Switch Case Action Subsystem/1(Out1) -> Merge/2
  Merge/1 -> [VTQD_CreepFinalSpd_kph]  "VTQD_CreepFinalSpd_kph"
  NOT/1 -> Logical Operator3/7
  NOT3/1 -> Logical Operator3/8
  [VTQD_OPDOn2Off_flg] -> NOT4/1
  NOT4/1 -> Logical Operator3/2
  [VTQD_CreepEnable_flg] -> If Action Subsystem1/9(VTQD_CreepEnable_flg)
  AND6/1 -> [VTQD_ActBPSPosnInRange_flg]  "VTQD_ActBPSPosnInRange_flg"
  [VTQD_ActBPSPosnInRange_flg] -> If Action Subsystem1/1(VTQD_ActBPSPosnInRange_flg)
  [VTQD_CreepErrSpd_kph] -> If Action Subsystem1/2(VTQD_CreepErrSpd_kph)
  [VTQD_CreepPterm_c] -> If Action Subsystem1/3(VTQD_CreepPterm_c)
  [VTQD_CreepIterm_c] -> If Action Subsystem1/4(VTQD_CreepIterm_c)
  task_time_s/1 -> [task_time_s]
  [VTQD_CreepDeltaTq_Nm] -> If Action Subsystem1/5(VTQD_CreepDeltaTq_Nm)
  [task_time_s] -> If Action Subsystem1/7(task_time_s)
  [VTQD_ActBPSPosn_pct] -> If Action Subsystem1/6(VTQD_ActBPSPosn_pct)
  If Action Subsystem1/1(VTQD_CreepTotalOfstTq_Nm) -> [VTQD_CreepTotalOfstTq_Nm]  "VTQD_CreepTotalOfstTq_Nm"
  [VTQD_CreepTotalOfstTq_Nm] -> Add2/2
  [VTQD_PedalMapWhlTq_Nm] -> GreaterThan/1
  [VTQD_CreepWhlTqDem_Nm] -> Unit Delay/1
  NOT15/1 -> AND15/1
  Constant63/1 -> Relational Operator5/2
  GreaterThan/1 -> AND15/2
  [VVMC_APSActive_flg] -> NOT15/1
  Unit Delay/1 -> GreaterThan/2
  [VTQD_ActAPSPosn_pct] -> Relational Operator5/1
  AND15/1 -> Switch15/3
  Relational Operator5/1 -> AND14/3
  Detect Increase/1 -> OR9/1
  Equal38/1 -> Detect Increase/1
  Constant64/1 -> Equal38/2
  [VTQD_RegenMode_enum] -> Equal38/1
  Detect Change/1 -> OR9/2
  OR9/1 -> OR1/13
  [VVMC_APSSpeedCMD_kph] -> Switch1/1
  [VVMC_APSSpeedCMD_kph] -> Switch2/1
  VTQD_ActAPSPosn_pct/1 -> [VTQD_ActAPSPosn_pct]
  [VVMC_CAASActive_flg] -> OR1/15
  Constant65/1 -> Equal39/2
  AND5/1 -> OR1/16
  Equal39/1 -> OR5/3
  [VVMC_APSReq_enum] -> Equal39/1
  Constant5/1 -> Equal20/2
  OR5/1 -> AND5/2
  [VVMC_APSSpeedCMD_kph] -> Relational Operator1/1
  [VVMC_APSActive_flg] -> AND5/1
  Relational Operator1/1 -> OR5/1
  Equal20/1 -> OR5/2
  Constant1/1 -> Relational Operator1/2
  [VVMC_APSReq_enum] -> Equal20/1
  VVMC_CAASActive_flg/1 -> [VVMC_CAASActive_flg]
  [VTQD_VehActSpd_kph] -> MTQD_CreepIterm_Z_Nm/1
  MTQD_CreepIterm_Z_Nm/1 -> [VTQD_CreepIterm_c]  "VTQD_CreepIterm_c"
  [VTQD_CreepErrSpd_kph] -> MTQD_CreepIterm_Z_Nm/2
  [VTQD_VehActSpd_kph] -> MTQD_CreepPreloadTime_Y_s/1

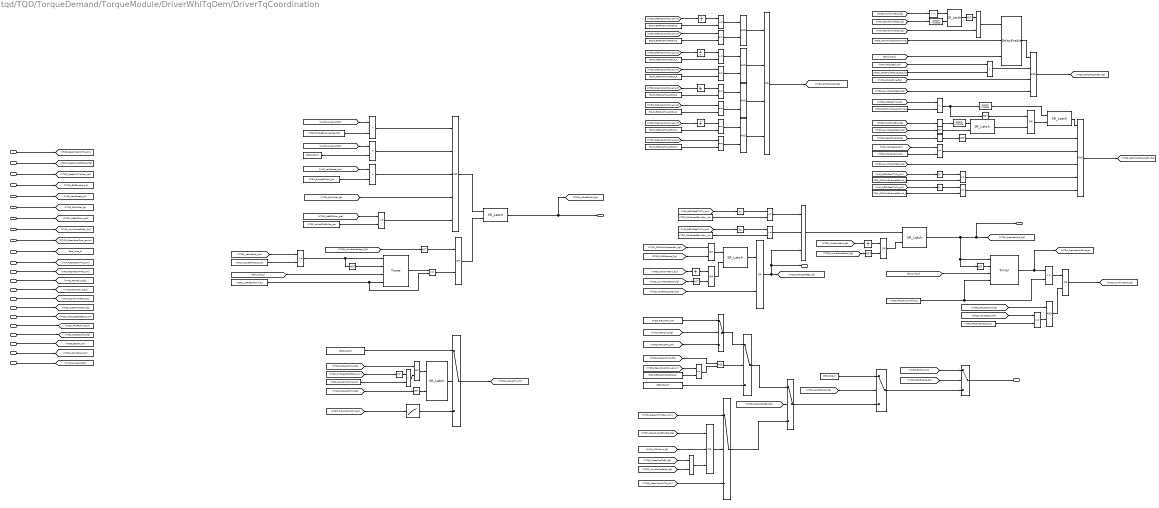
== system tqd/TQD/TorqueDemand/TorqueModule/DriverWhlTqDem/DriverTqCoordination ==
  VTQD_PedalMapWhlTq_Nm : Inport
  VTQD_CreepPrLoadEnable_flg : Inport  Port=2
  VTQD_CreepWhlTqDem_Nm : Inport  Port=3
  VTQD_BOSEnable_flg : Inport  Port=4
  VINP_VehSpeed_kph : Inport  Port=5
  VTQD_BrkSwSta_flg : Inport  Port=6
  VTQD_ActBPSPosn_pct : Inport  Port=7
  VTQD_LowIdleAccPedal_flg : Inport  Port=8
  VTQD_GearActualPosn_enum : Inport  Port=9
  task_time_s : Inport  Port=10
  VINP_FrEDURealTMTq_Nm : Inport  Port=11
  VINP_RrEDURealTMTq_Nm : Inport  Port=12
  VVMC_APSActive_flg : Inport  Port=13
  VVMC_ADASActive_flg : Inport  Port=14
  VINP_ACCVehHoldReq_flg : Inport  Port=15
  VTQD_CreepProtTqEn_flg : Inport  Port=16
  VTQD_TqTargetShaftSpd_rpm : Inport  Port=17
  VTQD_APSReqTimer_s : Inport  Port=18
  VTQD_CreepEnable_flg : Inport  Port=19
  VTQD_BOSTq_Nm : Inport  Port=20
  VTQD_VehActSpd_kph : Inport  Port=21
  VVMC_LongAcc_Gps : Inport  Port=22
  AND : Logic  Inputs=3  AllPortsSameDT=off  OutDataTypeStr=boolean
  AND{1..3,7..11} (8 alike) : Logic  AllPortsSameDT=off  OutDataTypeStr=boolean
  AND4 : Logic  Inputs=6  AllPortsSameDT=off  OutDataTypeStr=boolean
  AND5 : Logic  Inputs=4  AllPortsSameDT=off  OutDataTypeStr=boolean
  AND6 : Logic  Inputs=5  AllPortsSameDT=off  OutDataTypeStr=boolean
  Abs{,1..4} (5 alike) : Abs
  Constant : Constant  Value=KTQD_LoSpdCtrlBrkPos_pct
  Constant1 : Constant  Value=KTQD_RrPreLoadBoundary_Nm
  Constant{2,10,15,17} (4 alike) : Constant  Value=ZERO_FLOAT
  Constant11 : Constant  Value=KTQD_ADASHoldPreLoadspd_kph
  Constant12 : Constant  Value=KTQD_ADASHoldDelayEnTime_s
  Constant13 : Constant  Value=KTQD_EmergBrkSpd_kph
  Constant14 : Constant  Value=KTQD_EmergBrkLongAccel_Gps
  Constant16 : Constant  Value=KTQD_PreLoadTqHold_rpm
  Constant18 : Constant  Value=KTQD_OPDHoldPreLoadTime_s
  Constant19 : Constant  Value=KTQD_PreLoad_Holdtime_s
  Constant20 : Constant  Value=KTQD_APSZeroSpd_kph
  Constant21 : Constant  Value=ENUM_GEARACTUALPOSN_D
  Constant22 : Constant  Value=ENUM_GEARACTUALPOSN_D
  Constant{4,6,23..24} (4 alike) : Constant  Value=ENUM_GEARACTUALPOSN_R
  Constant25 : Constant  Value=KTQD_LoSPdBrkRlsTime_s
  Constant26 : Constant  Value=KTQD_LoSpdBrkRlsSpd_kph
  Constant27 : Constant  Value=KTQD_OPDHoldPreLoadBound_Nm
  Constant28 : Constant  Value=KTQD_OPDHoldPreLoadBound_Nm
  Constant29 : Constant  Value=KTQD_PreLoadDisSpd_kph
  Constant3 : Constant  Value=KTQD_RrPreLoadBoundary_Nm
  Constant5 : Constant  Value=ENUM_GEARACTUALPOSN_N
  Constant7 : Constant  Value=ENUM_GEARACTUALPOSN_P
  Constant8 : Constant  Value=ENUM_GEARACTUALPOSN_P
  Constant9 : Constant  Value=KTQD_PreLoadTq_Nm
  Delay : Delay  DelayLength=1
  Delay1 : Delay  DelayLength=1
  Delay2 : Delay  DelayLength=1
  DelayEnable : hcu_lib/Basic_Blocks/DelayEnable
  Detect Increase : simulink/Logic and Bit Operations/Detect Increase  vinit=0.0  OutDataTypeStr=boolean
  Detect Increase1 : simulink/Logic and Bit Operations/Detect Increase  vinit=0.0  OutDataTypeStr=boolean
  Detect Increase2 : simulink/Logic and Bit Operations/Detect Increase  vinit=0.0  OutDataTypeStr=boolean
  Equal{1..4,6,8} (6 alike) : RelationalOperator  Operator===  OutDataTypeStr=boolean  RndMeth=Simplest
  Equal5 : RelationalOperator  Operator=~=  OutDataTypeStr=boolean  RndMeth=Simplest
  Equal7 : RelationalOperator  Operator=~=  OutDataTypeStr=boolean  RndMeth=Simplest
  Equal9 : RelationalOperator  Operator=~=  OutDataTypeStr=boolean  RndMeth=Simplest
  GreaterThan : RelationalOperator  OutDataTypeStr=boolean  RndMeth=Simplest
  Logical Operator : Logic  AllPortsSameDT=off  OutDataTypeStr=boolean
  MTQD_PreLoadTq_Y_Nm1 : Lookup_n-D  NumberOfTableDimensions=1  BreakpointsForDimension1=ATQD_PreLoadTq_X_s  Table=MTQD_PreLoadTq_Y_Nm  ExtrapMethod=Clip  InternalRulePriority=Speed  RndMeth=Simplest  InputSameDT=on
  NOT{,1..9} (10 alike) : Logic  Operator=NOT  AllPortsSameDT=off  OutDataTypeStr=boolean
  OR : Logic  Operator=OR  Inputs=3  AllPortsSameDT=off  OutDataTypeStr=boolean
  OR{1..2,4..8} (7 alike) : Logic  Operator=OR  AllPortsSameDT=off  OutDataTypeStr=boolean
  OR3 : Logic  Operator=OR  Inputs=4  AllPortsSameDT=off  OutDataTypeStr=boolean
  Relational Operator : RelationalOperator  OutDataTypeStr=boolean  RndMeth=Simplest
  Relational Operator{1..2,6,11..14} (7 alike) : RelationalOperator  Operator=<=  OutDataTypeStr=boolean  RndMeth=Simplest
  Relational Operator{3,8..10} (4 alike) : RelationalOperator  Operator=<  OutDataTypeStr=boolean  RndMeth=Simplest
  Relational Operator4 : RelationalOperator  Operator=>  OutDataTypeStr=boolean  RndMeth=Simplest
  Relational Operator5 : RelationalOperator  Operator=>  OutDataTypeStr=boolean  RndMeth=Simplest
  Relational Operator7 : RelationalOperator  OutDataTypeStr=boolean  RndMeth=Simplest
  SR_Latch{,1..6} (7 alike) : hcu_lib/Basic_Blocks/SR_Latch
  Switch{,1..4} (5 alike) : Switch  Criteria=u2 ~= 0
      Switch1 settings: AttributesFormatString=<%<Criteria>>
      Switch2 settings: AttributesFormatString=<%<Criteria>>
  Switch5 : Switch  Criteria=u2 > Threshold
  Switch6 : Switch  Criteria=u2 > Threshold
  Timer : hcu_lib/Basic_Blocks/Timer
  Timer1 : hcu_lib/Basic_Blocks/Timer
  Unit Delay{1..6} (6 alike) : UnitDelay  SampleTime=-1  HasFrameUpgradeWarning=on
  VTQD_DriverWhlTqDem_Nm : Outport
  VTQD_LoSpdBrkCtrl_flg : Outport  Port=2
  VTQD_PreLoadHold_flg : Outport  Port=3
  VTQD_PreLoadPreEn_flg : Outport  Port=4
  wires:
  VTQD_PedalMapWhlTq_Nm/1 -> [VTQD_PedalMapWhlTq_Nm]
  VTQD_CreepPrLoadEnable_flg/1 -> [VTQD_CreepPrLoadEnable_flg]
  VTQD_CreepWhlTqDem_Nm/1 -> [VTQD_CreepWhlTqDem_Nm]
  VTQD_BOSEnable_flg/1 -> [VTQD_BOSEnable_flg]
  [VTQD_BOSEnable_flg] -> Switch1/2
  [VTQD_PedalMapWhlTq_Nm] -> Switch2/3
  [VTQD_CreepWhlTqDem_Nm] -> Switch2/1
  [VTQD_ActBPSPosn_pct] -> Relational Operator/1
  Constant/1 -> Relational Operator/2
  SR_Latch/1 -> [VTQD_LoSpdBrkCtrl_flg], VTQD_LoSpdBrkCtrl_flg/1  "VTQD_LoSpdBrkCtrl_flg"
  Constant10/1 -> Switch/1
  Switch1/1 -> VTQD_DriverWhlTqDem_Nm/1  "VTQD_DriverWhlTqDem_Nm"
  Switch/1 -> Switch1/3
  [VTQD_LowIdleAccPedal_flg] -> NOT/1
  Constant26/1 -> Relational Operator6/2
  Relational Operator6/1 -> Timer/1, NOT1/1
  Timer/1 -> Relational Operator7/1
  NOT/1 -> OR2/1
  Relational Operator7/1 -> OR2/2
  OR2/1 -> SR_Latch/2  "VTQD_LoBrkCtrlReset_flg"
  NOT1/1 -> Timer/2
  Constant13/1 -> Relational Operator10/2
  [VINP_VehSpeed_kph] -> Relational Operator10/1
  Constant15/1 -> Relational Operator9/2
  [VVMC_LongAcc_Gps] -> Relational Operator9/1
  Constant14/1 -> Relational Operator8/2
  [VVMC_LongAcc_Gps] -> Relational Operator8/1
  Relational Operator10/1 -> AND6/3
  Relational Operator9/1 -> AND6/2
  Relational Operator8/1 -> AND6/1
  [task_time_s] -> Timer/3
  VINP_VehSpeed_kph/1 -> [VINP_VehSpeed_kph]
  VTQD_BrkSwSta_flg/1 -> [VTQD_BrkSwSta_flg]
  VTQD_ActBPSPosn_pct/1 -> [VTQD_ActBPSPosn_pct]
  VTQD_LowIdleAccPedal_flg/1 -> [VTQD_LowIdleAccPedal_flg]
  VTQD_GearActualPosn_enum/1 -> [VTQD_GearActualPosn_enum]
  task_time_s/1 -> [task_time_s]
  Constant25/1 -> Relational Operator7/2, Timer/4
  AND6/1 -> SR_Latch/1  "VTQD_TestLoSpdBrkCtrl_flg"
  [VTQD_BrkSwSta_flg] -> AND6/4
  Relational Operator/1 -> AND6/5
  Timer1/1 -> [VTQD_PreLoadHoldtime_s], GreaterThan/1  "VTQD_PreLoadHoldtime_s"
  [VTQD_PreLoadPreEn_flg] -> Switch4/2
  [VTQD_HoldtimeEnd_flg] -> Unit Delay4/1
  Constant19/1 -> Timer1/4, GreaterThan/2
  [task_time_s] -> Timer1/3
  Unit Delay2/1 -> Equal5/1
  [VTQD_GearActualPosn_enum] -> Unit Delay2/1
  Constant23/1 -> Equal7/2
  [VTQD_GearActualPosn_enum] -> Equal8/1
  Equal5/1 -> AND8/1
  AND9/1 -> OR3/2
  Constant21/1 -> Equal5/2
  Constant24/1 -> Equal8/2
  Unit Delay3/1 -> Equal7/1
  Constant22/1 -> Equal6/2
  AND8/1 -> OR3/1
  [VTQD_GearActualPosn_enum] -> Unit Delay3/1
  [VTQD_GearActualPosn_enum] -> Equal6/1
  Equal6/1 -> AND8/2
  Equal8/1 -> AND9/2
  OR3/1 -> [VTQD_ShiftPreload_flg]  "VTQD_ShiftPreload_flg"
  Equal7/1 -> AND9/1
  NOT2/1 -> Timer1/2
  Unit Delay4/1 -> OR4/1
  OR4/1 -> SR_Latch1/2
  Switch2/1 -> Switch4/3
  Switch4/1 -> Switch/3
  [VTQD_LowIdleAccPedal_flg] -> NOT3/1
  NOT3/1 -> OR4/2
  [VTQD_LoSpdBrkCtrl_flg] -> Switch/2
  VINP_FrEDURealTMTq_Nm/1 -> [VINP_FrEDURealTMTq_Nm]
  VINP_RrEDURealTMTq_Nm/1 -> [VINP_RrEDURealTMTq_Nm]
  [VTQD_GearActualPosn_enum] -> Equal2/1
  Constant5/1 -> Equal2/2
  Equal2/1 -> AND1/2
  Equal1/1 -> AND1/1
  Constant4/1 -> Equal1/2
  AND1/1 -> OR3/3
  [VTQD_GearActualPosn_enum] -> Unit Delay1/1
  Unit Delay1/1 -> Equal1/1
  Constant3/1 -> Relational Operator2/2
  Relational Operator2/1 -> AND/1
  Constant1/1 -> Relational Operator1/2
  Abs1/1 -> Relational Operator2/1
  Relational Operator1/1 -> AND/2
  Abs/1 -> Relational Operator1/1
  [VINP_RrEDURealTMTq_Nm] -> Abs/1
  [VINP_FrEDURealTMTq_Nm] -> Abs1/1
  OR5/1 -> AND/3, VTQD_PreLoadPreEn_flg/1, [VTQD_PreLoadPreEn_flg]  "VTQD_PreLoadPreEn_flg"
  Switch3/1 -> Switch4/1
  Constant2/1 -> Switch3/3
  Unit Delay5/1 -> Equal3/1
  [VTQD_GearActualPosn_enum] -> Unit Delay5/1
  Constant6/1 -> Equal3/2
  Equal3/1 -> AND2/1
  Equal4/1 -> AND2/2
  Constant7/1 -> Equal4/2
  [VTQD_GearActualPosn_enum] -> Equal4/1
  AND2/1 -> OR3/4
  AND/1 -> SR_Latch2/1
  NOT4/1 -> OR1/2
  [VTQD_LowIdleAccPedal_flg] -> NOT4/1
  Unit Delay6/1 -> OR1/1
  [VTQD_HoldtimeEnd_flg] -> Unit Delay6/1
  OR1/1 -> SR_Latch2/2
  [VTQD_GearActualPosn_enum] -> Equal9/1
  Constant8/1 -> Equal9/2
  Logical Operator/1 -> Switch3/2
  [VTQD_PreLoadHold_flg] -> Logical Operator/1
  Equal9/1 -> Logical Operator/2
  SR_Latch2/1 -> VTQD_PreLoadHold_flg/1, [VTQD_PreLoadHold_flg], Timer1/1, NOT2/1  "VTQD_PreLoadHold_flg"
  Constant12/1 -> DelayEnable/2
  Relational Operator3/1 -> AND5/2
  Constant11/1 -> Relational Operator3/2
  AND5/1 -> [VTQD_ADASPreLoadEn_flg]  "VTQD_ADASPreLoadEn_flg"
  AND7/1 -> DelayEnable/1  "VTQD_ADASPreLoadHold_flg"
  [VVMC_ADASActive_flg] -> AND5/3
  [VINP_ACCVehHoldReq_flg] -> Detect Increase/1
  Delay/1 -> SR_Latch3/1
  DelayEnable/1 -> AND5/1
  [VTQD_HoldtimeEnd_flg] -> Delay/1
  SR_Latch3/1 -> NOT5/1
  [VINP_ACCVehHoldReq_flg] -> AND7/2
  Detect Increase/1 -> SR_Latch3/2
  [task_time_s] -> DelayEnable/3  "task_time_s"
  [VINP_VehSpeed_kph] -> Relational Operator3/1
  NOT5/1 -> AND7/1
  Constant9/1 -> Switch5/1
  [VVMC_APSActive_flg] -> Switch5/2
  Switch5/1 -> Switch3/1
  [VVMC_APSActive_flg] -> OR/2
  OR/1 -> Switch2/2
  [VTQD_CreepPrLoadEnable_flg] -> OR/1
  [VTQD_ADASPreLoadEn_flg] -> OR5/2
  SR_Latch1/1 -> OR5/1
  VVMC_APSActive_flg/1 -> [VVMC_APSActive_flg]
  VVMC_ADASActive_flg/1 -> [VVMC_ADASActive_flg]
  VINP_ACCVehHoldReq_flg/1 -> [VINP_ACCVehHoldReq_flg]
  VTQD_CreepProtTqEn_flg/1 -> [VTQD_CreepProtTqEn_flg]
  [VTQD_CreepProtTqEn_flg] -> AND10/1
  [VTQD_LowIdleAccPedal_flg] -> AND10/2
  AND10/1 -> OR/3
  [VTQD_LowIdleAccPedal_flg] -> AND5/4
  [VTQD_PreLoadHold_flg] -> AND3/1
  Constant17/1 -> Switch6/1
  Abs2/1 -> Relational Operator4/1
  [VTQD_PreLoadHold_flg] -> NOT6/1
  [VTQD_TqTargetShaftSpd_rpm] -> Abs2/1
  Constant16/1 -> Relational Operator4/2
  NOT6/1 -> SR_Latch4/2
  Switch6/1 -> [VTQD_PreloadTq_Nm]  "VTQD_PreloadTq_Nm"
  SR_Latch4/1 -> Switch6/2
  MTQD_PreLoadTq_Y_Nm1/1 -> Switch6/3
  Relational Operator4/1 -> AND3/2
  AND3/1 -> SR_Latch4/1
  [VTQD_PreLoadHoldtime_s] -> MTQD_PreLoadTq_Y_Nm1/1
  [VTQD_PreloadTq_Nm] -> Switch5/3
  VTQD_TqTargetShaftSpd_rpm/1 -> [VTQD_TqTargetShaftSpd_rpm]
  VTQD_APSReqTimer_s/1 -> [VTQD_APSReqTimer_s]
  VTQD_CreepEnable_flg/1 -> [VTQD_CreepEnable_flg]
  VTQD_VehActSpd_kph/1 -> [VTQD_VehActSpd_kph]
  VTQD_BOSTq_Nm/1 -> [VTQD_BOSTq_Nm]
  [VTQD_BOSTq_Nm] -> Switch1/1
  [VTQD_VehActSpd_kph] -> Relational Operator6/1
  Detect Increase1/1 -> SR_Latch5/1
  OR6/1 -> SR_Latch5/2
  [VINP_VehSpeed_kph] -> Relational Operator11/1
  Relational Operator5/1 -> Detect Increase1/1, NOT8/1
  Delay2/1 -> NOT7/1
  NOT9/1 -> SR_Latch6/2
  SR_Latch5/1 -> AND4/1
  [VTQD_HoldtimeEnd_flg] -> Delay1/1
  NOT7/1 -> AND4/2
  Constant27/1 -> Relational Operator12/2
  Delay1/1 -> Detect Increase2/1
  Abs3/1 -> Relational Operator12/1
  Constant28/1 -> Relational Operator13/2
  Detect Increase2/1 -> SR_Latch6/1
  Relational Operator12/1 -> AND4/6
  Relational Operator13/1 -> AND4/5
  Relational Operator11/1 -> AND4/3
  [VINP_FrEDURealTMTq_Nm] -> Abs4/1
  [VINP_RrEDURealTMTq_Nm] -> Abs3/1
  Constant20/1 -> Relational Operator11/2
  [VTQD_APSReqTimer_s] -> Relational Operator5/1
  [VTQD_LowIdleAccPedal_flg] -> AND4/4
  SR_Latch6/1 -> OR6/2  "VTQD_PreLoadHoldtimeEnd_flg"
  AND4/1 -> [VTQD_OPDHoldPreLoadEn_flg]  "VTQD_OPDHoldPreLoadEn_flg"
  Abs4/1 -> Relational Operator13/1
  Constant18/1 -> Relational Operator5/2
  [VTQD_CreepEnable_flg] -> Delay2/1
  [VTQD_LowIdleAccPedal_flg] -> NOT9/1
  NOT8/1 -> OR6/1
  VVMC_LongAcc_Gps/1 -> [VVMC_LongAcc_Gps]
  [VTQD_OPDHoldPreLoadEn_flg] -> OR7/1
  [VTQD_ShiftPreload_flg] -> OR7/2
  OR7/1 -> SR_Latch1/1
  [VTQD_PreLoadHold_flg] -> AND11/1
  [VTQD_VehActSpd_kph] -> Relational Operator14/1
  Relational Operator14/1 -> AND11/2
  Constant29/1 -> Relational Operator14/2
  GreaterThan/1 -> OR8/1
  AND11/1 -> OR8/2
  OR8/1 -> [VTQD_HoldtimeEnd_flg]  "VTQD_HoldtimeEnd_flg"
